simulink model "WindupIllustration"  (Simulink 10.3)
settings: Solver=VariableStepAuto  StartTime=0.0  StopTime=20  RelTol=1e-3
settings Model: Creator=Mertcan  LastModifiedBy=Mertcan
settings SolverCC: AlgebraicLoopSolver=Auto
settings DataIOCC: SaveFormat=Dataset  SignalLoggingSaveFormat=Dataset  ReturnWorkspaceOutputs=on
settings OptimizationCC: ExpressionDepthLimit=128  LifeSpan=auto
settings DebuggingCC: UnderspecifiedInitializationDetection=Simplified  MergeDetectMultiDrivingBlocksExec=error  FcnCallInpInsideContextMsg=error  StateNameClashWarn=none  SFUnexpectedBacktrackingDiag=error  SFNoUnconditionalDefaultTransitionDiag=error  SFExecutionAtInitializationDiag=warning  SFMachineParentedDataDiag=error  ArithmeticOperatorsInVariantConditions=error
settings HardwareCC: ProdBitPerPointer=64  ProdBitPerSizeT=64  ProdBitPerPtrDiffT=64  ProdLargestAtomicFloat=Float  ProdIntDivRoundTo=Zero  ProdEndianess=LittleEndian  ProdWordSize=64  ProdHWDeviceType=Intel->x86-64 (Windows64)
settings ModelReferenceCC: PropagateSignalLabelsOutOfModel=on
settings SFSimCC: SimUseLocalCustomCode=on  CustomCodeUndefinedFunction=FilterOut
settings RTWCC: RTWUseLocalCustomCode=on
settings CodeAppCC: StateflowObjectComments=off
settings GRTTargetCC: TargetLangStandard=C99 (ISO)  CombineOutputUpdateFcns=on  GRTInterface=off
settings ConfigComp: CovMetricSettings=dwe  CovSaveCumulativeToWorkspaceVar=off  CovSaveSingleToWorkspaceVar=off  CovExternalEMLEnable=on

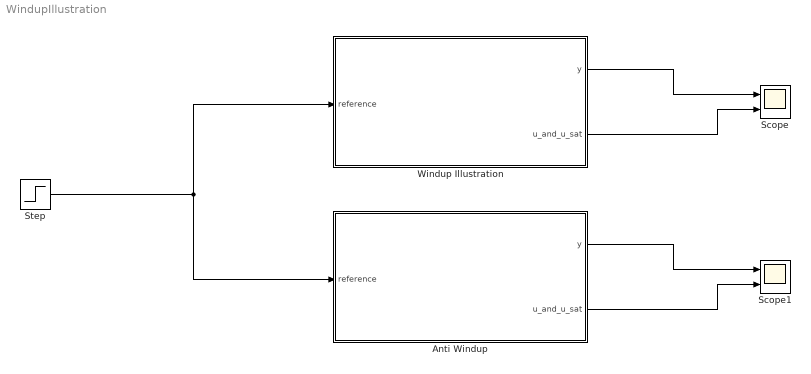
== system WindupIllustration ==
  Anti Windup : Subsystem
  Scope : Scope  NumInputPorts=2
  Scope1 : Scope  NumInputPorts=2
  Step : Step  Time=6  Before=1  After=0  SampleTime=0
  Windup Illustration : Subsystem
  wires:
  Windup Illustration/1(y) -> Scope/1
  Windup Illustration/2(u_and_u_sat) -> Scope/2
  Anti Windup/1(y) -> Scope1/1
  Anti Windup/2(u_and_u_sat) -> Scope1/2
  Step/1 -> Windup Illustration/1(reference), Anti Windup/1(reference)

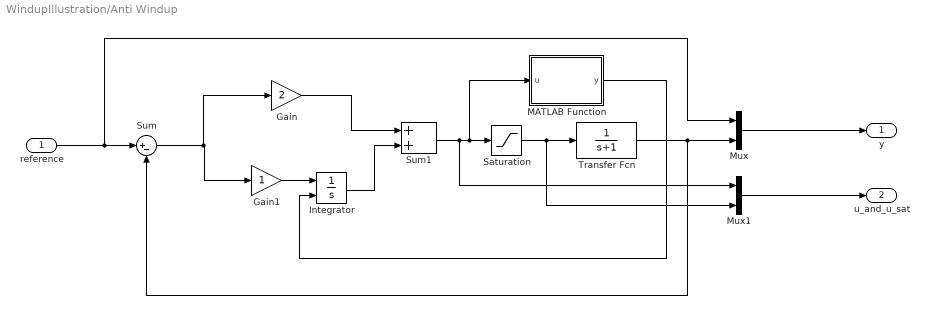
== system WindupIllustration/Anti Windup ==
  reference : Inport
  Gain : Gain  Gain=2
  Gain1 : Gain
  Integrator : Integrator  ExternalReset=level  UpperSaturationLimit=0.1  LowerSaturationLimit=-0.1
  MATLAB Function : MATLAB Function  TreatAsAtomicUnit=on
  Mux : Mux  Inputs=2
  Mux1 : Mux  Inputs=2
  Saturation : Saturate
  Sum : Sum  Inputs=|+-
  Sum1 : Sum
  Transfer Fcn : TransferFcn  Denominator=[1 1]
  y : Outport
  u_and_u_sat : Outport  Port=2
  wires:
  Mux1/1 -> u_and_u_sat/1
  Mux/1 -> y/1
  Sum/1 -> Gain/1, Gain1/1
  Transfer Fcn/1 -> Mux/2, Sum/2
  Gain/1 -> Sum1/1
  Saturation/1 -> Mux1/2, Transfer Fcn/1
  Integrator/1 -> Sum1/2
  Gain1/1 -> Integrator/1
  Sum1/1 -> Mux1/1, MATLAB Function/1(u), Saturation/1
  reference/1 -> Mux/1, Sum/1
  MATLAB Function/1(y) -> Integrator/2

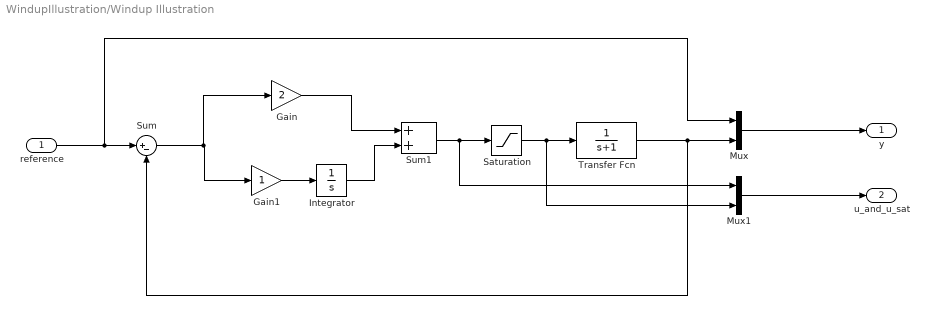
== system WindupIllustration/Windup Illustration ==
  reference : Inport
  Gain : Gain  Gain=2
  Gain1 : Gain
  Integrator : Integrator  UpperSaturationLimit=0.1  LowerSaturationLimit=-0.1
  Mux : Mux  Inputs=2
  Mux1 : Mux  Inputs=2
  Saturation : Saturate
  Sum : Sum  Inputs=|+-
  Sum1 : Sum
  Transfer Fcn : TransferFcn  Denominator=[1 1]
  y : Outport
  u_and_u_sat : Outport  Port=2
  wires:
  reference/1 -> Sum/1, Mux/1
  Sum1/1 -> Saturation/1, Mux1/1
  Gain1/1 -> Integrator/1
  Integrator/1 -> Sum1/2
  Saturation/1 -> Transfer Fcn/1, Mux1/2
  Gain/1 -> Sum1/1
  Transfer Fcn/1 -> Sum/2, Mux/2
  Sum/1 -> Gain1/1, Gain/1
  Mux/1 -> y/1
  Mux1/1 -> u_and_u_sat/1

== matlab function Anti Windup/MATLAB Function ==
  data: u input double; y output double
function y = fcn(u)
if u >= 0.5
    y = 1;
else
    y = 0;
end
